simulink model "fig8_10a"  (R2013a)
settings: Solver=ode45  SolverMode=SingleTasking  StartTime=0.0  StopTime=2  RelTol=1e-3  AbsTol=1e-6
libraries: simulink x2
settings Model: ExtModeTrigMode=oneshot  ExtModeArmWhenConnect=off  Creator=David Powell  LastModifiedBy=David Powell
settings DataIOCC: LimitDataPoints=off  SignalLoggingSaveFormat=ModelDataLogs
settings OptimizationCC: BlockReduction=off  BooleanDataType=off
settings DebuggingCC: SaveWithParameterizedLinksMsg=none  SignalResolutionControl=TryResolveAllWithWarning  SolverPrmCheckMsg=none  MultiTaskDSMMsg=warning  MultiTaskCondExecSysMsg=none  StrictBusMsg=None
settings HardwareCC: TargetUnknown=on
settings RTWCC: IncludeERTFirstTime=on
settings GRTTargetCC: CombineOutputUpdateFcns=off  GRTInterface=on

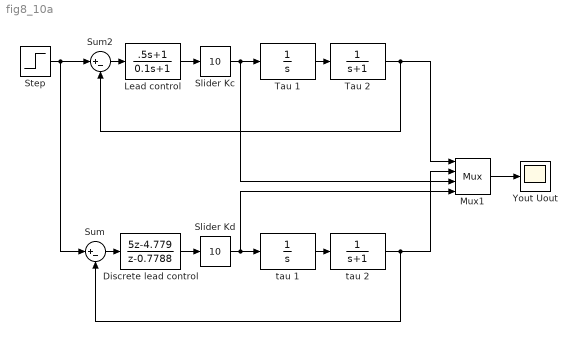
== system fig8_10a ==
  Discrete lead control : DiscreteTransferFcn  Numerator="[5  -4.779]"  Denominator=[1 -0.7788]  SampleTime=.025
  Lead control : TransferFcn  Numerator=[.5 1]  Denominator=[0.1 1]
  Mux1 : Mux
  Slider Kc : simulink/Math Operations/Slider Gain  low=0  gain=10  high=20
  Slider Kd : simulink/Math Operations/Slider Gain  low=0  gain=10  high=20
  Step : Step  Time=0  SampleTime=.001
  Sum : Sum  Inputs=|+-  InputSameDT=on  OutDataTypeStr=Inherit: Same as first input
  Sum2 : Sum  Inputs=|+-  InputSameDT=on  OutDataTypeStr=Inherit: Same as first input
  Tau 1 : TransferFcn  Numerator=1  Denominator=[1 0]
  Tau 2 : TransferFcn  Numerator=1  Denominator=[1 1]
  Yout Uout : Scope
      settings: Tag=position  TickLabels=on  SaveName=ycd
  tau 1 : TransferFcn  Numerator=1  Denominator=[1 0]
  tau 2 : TransferFcn  Numerator=1  Denominator=[1 1]
  wires:
  Lead control/1 -> Slider Kc/1
  Sum2/1 -> Lead control/1
  Tau 1/1 -> Tau 2/1
  Discrete lead control/1 -> Slider Kd/1
  tau 1/1 -> tau 2/1
  Step/1 -> Sum2/1, Sum/1
  Tau 2/1 -> Mux1/1, Sum2/2
  Sum/1 -> Discrete lead control/1
  tau 2/1 -> Mux1/2, Sum/2
  Slider Kd/1 -> tau 1/1, Mux1/4
  Mux1/1 -> Yout Uout/1
  Slider Kc/1 -> Tau 1/1, Mux1/3
